simulink library "lib_utils"  (R2025a)
settings: Solver=VariableStepAuto  StartTime=0.0  StopTime=10.0  RelTol=1e-3
undefined symbols (not defined in the file or in its folder): IAU, params
libraries: aerolibtransform2 x1
settings Model: Creator=Blind  LastModifiedBy=Blind

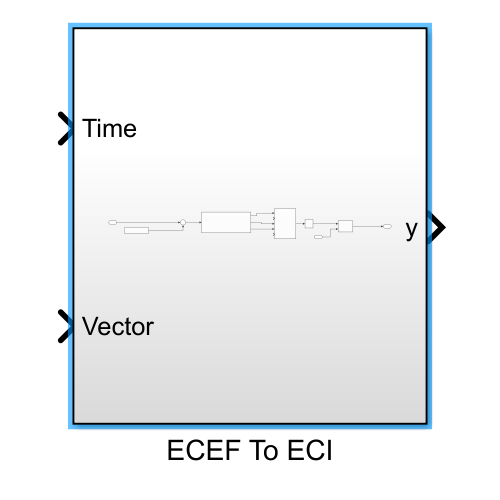
[thumbnail: Simulink's stored preview of the top-level diagram]
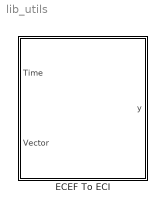
== system lib_utils ==
  ECEF To ECI : Subsystem

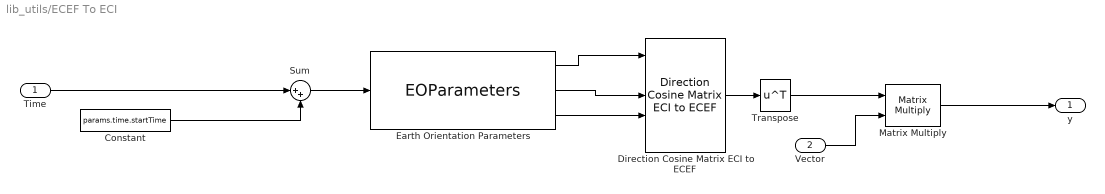
== system lib_utils/ECEF To ECI ==
  Time : Inport
  Vector : Inport  Port=2
  Constant : Constant  Value=params.time.startTime
  Direction Cosine Matrix ECI to ECEF : aerolibtransform2/Direction Cosine Matrix ECI to ECEF  red=IAU-2000/2006  year=2013  month=January  day=1  hour=0  min=0  sec=0  deltaT=Day  errorflag=Error  extraparamflag=on
      settings: AttributesFormatString=%<red>
  Earth Orientation Parameters : EOParameters
  Matrix Multiply : Product  Multiplication=Matrix(*)
  Sum : Sum  Inputs=|++
  Transpose : Math  Operator=transpose
  y : Outport
  wires:
  Earth Orientation Parameters/1 -> Direction Cosine Matrix ECI to ECEF/1
  Earth Orientation Parameters/2 -> Direction Cosine Matrix ECI to ECEF/3
  Earth Orientation Parameters/3 -> Direction Cosine Matrix ECI to ECEF/4
  Sum/1 -> Earth Orientation Parameters/1
  Time/1 -> Sum/1
  Constant/1 -> Sum/2
  Direction Cosine Matrix ECI to ECEF/1 -> Transpose/1
  Transpose/1 -> Matrix Multiply/1
  Vector/1 -> Matrix Multiply/2
  Matrix Multiply/1 -> y/1
